simulink model "sldemo_hardstop"  (R2019b)
settings: Solver=ode45  StartTime=0.0  StopTime=2.0  RelTol=1e-6  AbsTol=1e-6
StartFcn:
  | set_param('sldemo_hardstop/Scope','Open','on');
Description:
  | Friction Model with Hard Stops
  | 
  | This example shows how to model friction one way in Simulink(R). The two integrators in
  | the model calculate the velocity and position of the system, which is then used in
  | the Friction Model to calculate the friction force.
  | 
  | Running the simulation shows the initial condition response on the Scope.
settings Model: ExtModeTrigMode=oneshot  ExtModeArmWhenConnect=off  ExtModeAutoUpdateStatusClock=off  Creator=The MathWorks, Inc.  LastModifiedBy=The MathWorks, Inc.
settings SolverCC: AutoScaleAbsTol=off
settings DataIOCC: ExternalInput=[]  InitialState=[]  SaveFormat=StructureWithTime  SaveState=on  Refine=4
settings OptimizationCC: ExpressionDepthLimit=2147483647  InitFltsAndDblsToZero=on  LifeSpan=inf  BufferReusableBoundary=off
settings DebuggingCC: SaveWithParameterizedLinksMsg=none  UnderspecifiedInitializationDetection=Classic  MergeDetectMultiDrivingBlocksExec=none  SignalResolutionControl=TryResolveAllWithWarning  MultiTaskDSMMsg=warning  MultiTaskCondExecSysMsg=none  IntegerOverflowMsg=none  FcnCallInpInsideContextMsg=warning  BusObjectLabelMismatch=none  StateNameClashWarn=warning  SFUnexpectedBacktrackingDiag=warning  SFNoUnconditionalDefaultTransitionDiag=warning  SFExecutionAtInitializationDiag=none  IntegerSaturationMsg=none  ArithmeticOperatorsInVariantConditions=warning
settings HardwareCC: ProdBitPerPointer=32  ProdBitPerSizeT=32  ProdBitPerPtrDiffT=32  ProdLargestAtomicFloat=None  ProdIntDivRoundTo=Undefined  ProdEndianess=Unspecified  ProdWordSize=32  ProdHWDeviceType=32-bit Generic  TargetUnknown=on
settings ModelReferenceCC: PropagateSignalLabelsOutOfModel=off
settings SFSimCC: SimUseLocalCustomCode=off  CustomCodeUndefinedFunction=UseInterfaceOnly
settings RTWCC: Description=Generic Real-Time Target  RTWUseLocalCustomCode=off
settings CodeAppCC: StateflowObjectComments=on
settings GRTTargetCC: TargetFcnLib=ansi_tfl_tmw.mat  TargetLangStandard=C89/C90 (ANSI)  GeneratePreprocessorConditionals=Disable all  CombineOutputUpdateFcns=off  GRTInterface=on
settings ConfigComp: CovMetricSettings=dw  CovHtmlReporting=on  CovSaveCumulativeToWorkspaceVar=on  CovSaveSingleToWorkspaceVar=on  CovExternalEMLEnable=off  CovSFcnEnable=off

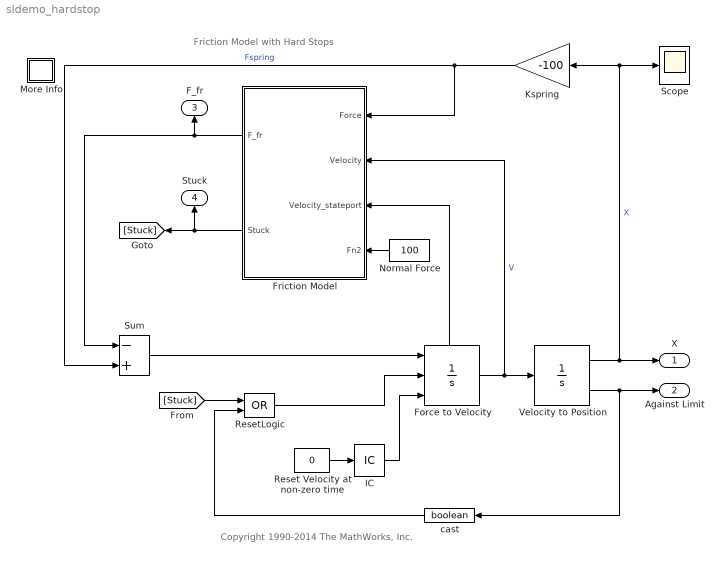
== system sldemo_hardstop ==
  note: Friction Model with Hard Stops
  note: Copyright 1990-2014 The MathWorks, Inc.
  Force to Velocity : Integrator  ExternalReset=rising  InitialConditionSource=external  ShowStatePort=on
  Friction Model : Subsystem
      mask Display:
      | port_label('input',1,'F (N)','texmode','on')
      | port_label('input',2,'Velocity (m/s)','texmode','on')
      | port_label('input',3,'VelState (m/s)','texmode','on')
      | port_label('input',4,'Fn (N)','texmode','on')
      | port_label('output',1,'Ff (N)','texmode','on')
      | port_label('output',2,'StuckFLAG','texmode','on')
  IC : InitialCondition  Value=100
  Kspring : Gain  Gain=-100  SaturateOnIntegerOverflow=on  OutDataTypeStr=Inherit: Same as input  ParamDataTypeStr=Inherit: Same as input
  More Info : Subsystem
      settings: OpenFcn=showExample('simulink_general/sldemo_hardstopExample')
      mask Display: disp('?')
  Normal Force : Constant  Value=100
  Reset Velocity at non-zero time : Constant  Value=0
  ResetLogic : Logic  Operator=OR  IconShape=distinctive  OutDataTypeStr=boolean
  Scope : Scope
  Sum : Sum  Inputs=-+  SaturateOnIntegerOverflow=on  InputSameDT=on  OutDataTypeStr=Inherit: Same as first input
  Velocity to Position : Integrator  InitialCondition=-0.5  LimitOutput=on  UpperSaturationLimit=5.5  LowerSaturationLimit=-3.5  ShowSaturationPort=on
      settings: AttributesFormatString=Xo = %<InitialCondition>
  cast : DataTypeConversion  OutDataTypeStr=boolean  SaturateOnIntegerOverflow=on  RndMeth=Zero
  X : Outport  InitialOutput=0  VectorParamsAs1DForOutWhenUnconnected=off
  Against Limit : Outport  Port=2  InitialOutput=0  VectorParamsAs1DForOutWhenUnconnected=off
  F_fr : Outport  Port=3  InitialOutput=0  VectorParamsAs1DForOutWhenUnconnected=off
  Stuck : Outport  Port=4  InitialOutput=0  VectorParamsAs1DForOutWhenUnconnected=off
  wires:
  Velocity to Position/1 -> X/1, Kspring/1, Scope/1  "X"
  Velocity to Position/2 -> cast/1, Against Limit/1
  Reset Velocity at non-zero time/1 -> IC/1
  Sum/1 -> Force to Velocity/1
  Force to Velocity/1 -> Velocity to Position/1, Friction Model/2(Velocity)  "V"
  Normal Force/1 -> Friction Model/4(Fn2)
  ResetLogic/1 -> Force to Velocity/2
  Friction Model/1(F_fr) -> Sum/1, F_fr/1
  Kspring/1 -> Sum/2, Friction Model/1(Force)  "Fspring"
  IC/1 -> Force to Velocity/3
  Friction Model/2(Stuck) -> [Stuck], Stuck/1
  cast/1 -> ResetLogic/2
  Force to Velocity/State -> Friction Model/3(Velocity_stateport)
  [Stuck] -> ResetLogic/1

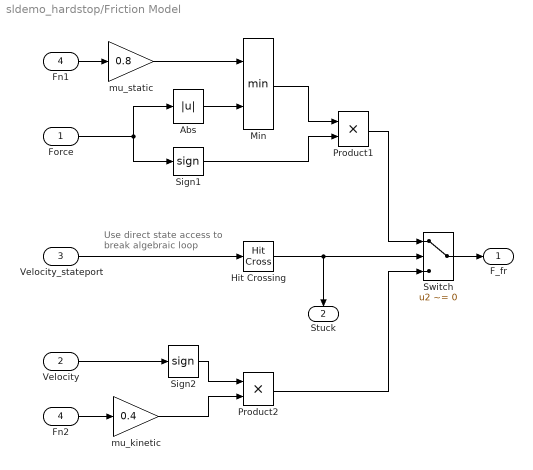
== system sldemo_hardstop/Friction Model ==
  note: Use direct state access to
      | break algebraic loop
  Force : Inport
  Velocity : Inport  Port=2
  Velocity_stateport : Inport  Port=3
  Fn2 : Inport  Port=4
  Abs : Abs  SaturateOnIntegerOverflow=on
  Fn1 : InportShadow  Port=4
  Hit Crossing : HitCross
  Min : MinMax  Inputs=2  SaturateOnIntegerOverflow=on  InputSameDT=on
  Product1 : Product  SaturateOnIntegerOverflow=on  InputSameDT=on  OutDataTypeStr=Inherit: Same as first input
  Product2 : Product  SaturateOnIntegerOverflow=on  InputSameDT=on  OutDataTypeStr=Inherit: Same as first input
  Sign1 : Signum
  Sign2 : Signum
  Switch : Switch  Criteria=u2 ~= 0  Threshold=0.5  InputSameDT=on
  mu_kinetic : Gain  Gain=0.4
  mu_static : Gain  Gain=0.8
  F_fr : Outport  InitialOutput=0  VectorParamsAs1DForOutWhenUnconnected=off
  Stuck : Outport  Port=2  InitialOutput=0  VectorParamsAs1DForOutWhenUnconnected=off
  wires:
  Hit Crossing/1 -> Stuck/1, Switch/2
  Product2/1 -> Switch/3
  Fn2/1 -> mu_kinetic/1
  Velocity/1 -> Sign2/1
  Switch/1 -> F_fr/1
  Velocity_stateport/1 -> Hit Crossing/1
  Product1/1 -> Switch/1
  Force/1 -> Abs/1, Sign1/1
  Abs/1 -> Min/2
  Fn1/1 -> mu_static/1
  Min/1 -> Product1/1
  Sign1/1 -> Product1/2
  Sign2/1 -> Product2/1
  mu_static/1 -> Min/1
  mu_kinetic/1 -> Product2/2

== system sldemo_hardstop/More Info ==
